simulink model "Tarea1Simulacion"  (R2025a)
settings: Solver=VariableStepAuto  StartTime=0.0  StopTime=10  RelTol=1e-3
settings Model: Creator=440G5  LastModifiedBy=440G5

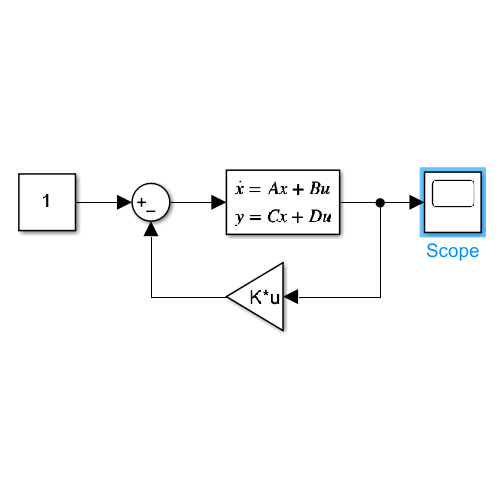
[thumbnail: Simulink's stored preview of the top-level diagram]
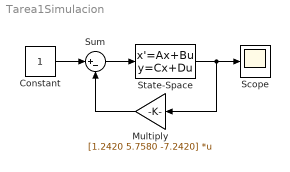
== system Tarea1Simulacion ==
  Constant : Constant
  Multiply : Gain  Gain=[1.2420 5.7580 -7.2420]  Multiplication=Matrix(K*u)
  Scope : Scope
      settings: ActiveDisplayYMinimum=-0.20599109855673844  ActiveDisplayYMaximum=0.18725323065049887
  State-Space : StateSpace  A=[0 1 0; 1 1 -1; 0 -1 0]  B=[1; 1; 0]  C=[1 0 0; 0 1 0; 0 0 1]  D=[0; 0; 0]  InitialCondition=[0 0 0]
  Sum : Sum  Inputs=|+-
  wires:
  State-Space/1 -> Multiply/1, Scope/1
  Constant/1 -> Sum/1
  Sum/1 -> State-Space/1
  Multiply/1 -> Sum/2
